simulink model "qp_sim"  (R2022a)
settings: Solver=VariableStepAuto  StartTime=0.0  StopTime=10.0  RelTol=1e-3
undefined symbols (not defined in the file): a1, a2, B, dq0, dtheta0, K, Kbar, Kp, Kv, m1, m2, q0, r_d, S, theta0
settings Model: Creator=mathe  LastModifiedBy=mathe

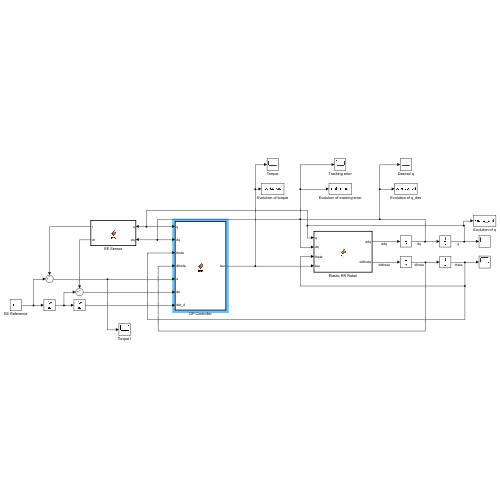
[thumbnail: Simulink's stored preview of the top-level diagram]
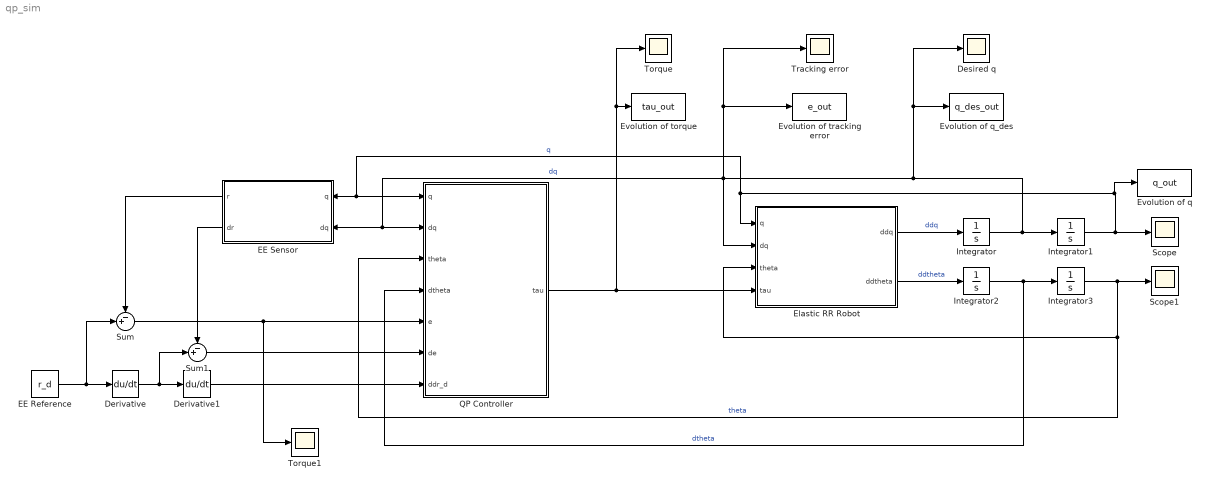
== system qp_sim ==
  Derivative : Derivative
  Derivative1 : Derivative
  Desired q : Scope
  EE Reference : Constant  Value=r_d
  EE Sensor : MATLAB Function  TreatAsAtomicUnit=on
  Elastic RR Robot : MATLAB Function  TreatAsAtomicUnit=on
  Evolution of q : ToWorkspace  VariableName=q_out  SaveFormat=Timeseries  SampleTime=-1
  Evolution of q_des : ToWorkspace  VariableName=q_des_out  SaveFormat=Timeseries  SampleTime=-1
  Evolution of torque : ToWorkspace  VariableName=tau_out  SaveFormat=Timeseries  SampleTime=-1
  Evolution of tracking error : ToWorkspace  VariableName=e_out  SaveFormat=Timeseries  SampleTime=-1
  Integrator : Integrator  InitialCondition=dq0
  Integrator1 : Integrator  InitialCondition=q0
  Integrator2 : Integrator  InitialCondition=dtheta0
  Integrator3 : Integrator  InitialCondition=theta0
  QP Controller : MATLAB Function  TreatAsAtomicUnit=on
  Scope : Scope
  Scope1 : Scope
  Sum : Sum  Inputs=-+|
  Sum1 : Sum  Inputs=-+|
  Torque : Scope
  Torque1 : Scope
  Tracking error : Scope
  wires:
  Elastic RR Robot/1(ddq) -> Integrator/1  "ddq"
  Integrator/1 -> Integrator1/1, Evolution of q_des/1, Desired q/1, EE Sensor/2(dq), QP Controller/2(dq), Elastic RR Robot/2(dq), Tracking error/1, Evolution of tracking error/1  "dq"
  Integrator2/1 -> QP Controller/4(dtheta), Integrator3/1  "dtheta"
  Elastic RR Robot/2(ddtheta) -> Integrator2/1  "ddtheta"
  Integrator3/1 -> Scope1/1, QP Controller/3(theta), Elastic RR Robot/3(theta)  "theta"
  Integrator1/1 -> QP Controller/1(q), EE Sensor/1(q), Elastic RR Robot/1(q), Evolution of q/1, Scope/1  "q"
  QP Controller/1(tau) -> Torque/1, Evolution of torque/1, Elastic RR Robot/4(tau)
  EE Reference/1 -> Sum/2, Derivative/1
  Derivative/1 -> Sum1/2, Derivative1/1
  Derivative1/1 -> QP Controller/7(ddr_d)
  EE Sensor/1(r) -> Sum/1
  EE Sensor/2(dr) -> Sum1/1
  Sum1/1 -> QP Controller/6(de)
  Sum/1 -> Torque1/1, QP Controller/5(e)

== matlab function qp_sim/QP Controller ==
  data: q input; tau output; dq input; theta input; dtheta input; e input; de input; ddr_d input; Kbar parameter; B parameter; S parameter; m1 parameter; m2 parameter; a1 parameter; a2 parameter; Kp parameter; Kv parameter
function tau  = fcn(q, dq, theta, dtheta, e, de, ddr_d, Kbar, B, S, ...
    m1, m2, a1, a2, Kp, Kv)

% Variable size for codegen
coder.varsize('x_star');

% Dynamic and Kinematic Matrices
[p, J, dJ] = kinematics(q, dq, a1, a2);
[M, C, G] = dynamics(q, dq, m1, m2, a1, a2);

% Getting Sizes
n = 2;
nj = 2;
m = 2;

% T1: Dynamics Compensation
A1 = [M, zeros(n,nj);
    zeros(nj,nj), B];
A1 = [A1, [zeros(nj,nj); -S.']]; 	% Required for proper concatenation.

b1 = Kbar*[q; theta] - blkdiag(C, zeros(nj,n))*[dq; dtheta] - [G; zeros(nj,1)];

% T2: Constraint Compliance
A2 = [J, zeros(m,nj), zeros(m,nj)];
b2 = -dJ*dq + ddr_d + Kp*e + Kv*de;

% T: Stack of Tasks
A = {A1, A2};
b = {b1, b2};

% Hierarchical QP
x_star = zeros(6,1);
x_star = hierarchical_qp_solve_active_set(A, b);

% Optimal Torque
tau = zeros(2,1);
tau = x_star(5:6,1);

== matlab function qp_sim/Elastic RR Robot ==
  data: q input; ddq output; dq input; theta input; tau input; ddtheta output; K parameter; B parameter; S parameter; m1 parameter; m2 parameter; a1 parameter; a2 parameter
function [ddq, ddtheta] = fcn(q, dq, theta, tau, K, B, S, m1, m2, a1, a2)

% Compute dynamic matrices
[M, C, G] = dynamics(q, dq, m1, m2, a1, a2);

% State evolutions
ddq = M\(S.'*K*(theta - q) - C*dq - G);
ddtheta = B\(tau - K*(theta - q));

== matlab function qp_sim/EE Sensor ==
  data: q input; dq input; r output; a2 parameter; a1 parameter; dr output
function [r, dr] = fcn(q, dq, a2, a1)

[r, J, ~] = kinematics(q, dq, a1, a2);
dr = J*dq;
